simulink model "Marine_LocoMotive_UAV_est_git"  (R2018a)
settings: Solver=ode4  StartTime=0.0  StopTime=40  FixedStep=T  MaxStep=2*T  MinStep=T  RelTol=1e-4
values from neighbouring files (symbols this model uses):
  a_11 = 0.05*m_b    (= 0.625)    [Marine_LocoMotive_UAV_est_git_parameters.m]    (also in Marine_LocoMotive_UAV_medium_est_git_parameters.m = 1.6875; heave_dynamics_chart.m)
  a_33 = m_b    (= 12.5)    [Marine_LocoMotive_UAV_est_git_parameters.m]    (also in Marine_LocoMotive_UAV_medium_est_git_parameters.m = 33.75; heave_dynamics_chart.m)
  A_w = 1*3.3/2    (= 1.65)    [Marine_LocoMotive_UAV_est_git_parameters.m]    (also in Marine_LocoMotive_UAV_medium_est_git_parameters.m = 0.6)
  A_w2 = 1*1.2/2    (= 0.6)    [Marine_LocoMotive_UAV_est_git_parameters.m]    (also in Marine_LocoMotive_UAV_medium_est_git_parameters.m = 0.305)
  Ac = 0.0331    [Marine_LocoMotive_UAV_est_git_parameters.m]    (also in Marine_LocoMotive_UAV_medium_est_git_parameters.m = 0.422)
  alpha_bar = pi/4    (= 0.785398163397)    [Marine_LocoMotive_UAV_est_git_parameters.m]    (also in Marine_LocoMotive_UAV_medium_est_git_parameters.m; heave_dynamics_chart.m = pi/4*sign(V_bar(j)))
  Am = sysd.denominator{1}    [Marine_LocoMotive_UAV_est_git_parameters.m]    (also in Marine_LocoMotive_UAV_medium_est_git_parameters.m)
  Am1_LPF = sysd.denominator{1}    [Marine_LocoMotive_UAV_est_git_parameters.m]    (also in Marine_LocoMotive_UAV_medium_est_git_parameters.m)
  Am2_LPF = sysd.denominator{1}    [Marine_LocoMotive_UAV_est_git_parameters.m]    (also in Marine_LocoMotive_UAV_medium_est_git_parameters.m)
  Am_asw_LPF = sysd.denominator{1}    [Marine_LocoMotive_UAV_est_git_parameters.m]    (also in Marine_LocoMotive_UAV_medium_est_git_parameters.m)
  Am_coup_LPF = sysd.denominator{1}    [Marine_LocoMotive_UAV_est_git_parameters.m]    (also in Marine_LocoMotive_UAV_medium_est_git_parameters.m)
  Am_fast_coup_LPF = sysd.denominator{1}    [Marine_LocoMotive_UAV_est_git_parameters.m]    (also in Marine_LocoMotive_UAV_medium_est_git_parameters.m)
  Am_rdeL_LPF = sysd.denominator{1}    [Marine_LocoMotive_UAV_est_git_parameters.m]    (also in Marine_LocoMotive_UAV_medium_est_git_parameters.m)
  Am_reL_LPF = sysd.denominator{1}    [Marine_LocoMotive_UAV_est_git_parameters.m]    (also in Marine_LocoMotive_UAV_medium_est_git_parameters.m)
  Am_rref20_LPF = sysd.denominator{1}    [Marine_LocoMotive_UAV_est_git_parameters.m]    (also in Marine_LocoMotive_UAV_medium_est_git_parameters.m)
  Am_rref_LPF = sysd.denominator{1}    [Marine_LocoMotive_UAV_est_git_parameters.m]    (also in Marine_LocoMotive_UAV_medium_est_git_parameters.m)
  AmAlpha_LPF = sysd.denominator{1}    [Marine_LocoMotive_UAV_est_git_parameters.m]    (also in Marine_LocoMotive_UAV_medium_est_git_parameters.m)
  Amp_sf = 3    [Marine_LocoMotive_UAV_est_git_parameters.m]    (also in Marine_LocoMotive_UAV_medium_est_git_parameters.m)
  Amp_sf_rp = 0.05*m_u*g    (= 0.8829)    [Marine_LocoMotive_UAV_est_git_parameters.m]    (also in Marine_LocoMotive_UAV_medium_est_git_parameters.m = 9.56475)
  AmV_LPF = sysd.denominator{1}    [Marine_LocoMotive_UAV_est_git_parameters.m]    (also in Marine_LocoMotive_UAV_medium_est_git_parameters.m)
  AmZ_LPF = sysd.denominator{1}    [Marine_LocoMotive_UAV_est_git_parameters.m]    (also in Marine_LocoMotive_UAV_medium_est_git_parameters.m)
  b_11 = 0    [Marine_LocoMotive_UAV_est_git_parameters.m]    (also in Marine_LocoMotive_UAV_medium_est_git_parameters.m; heave_dynamics_chart.m)
  b_33 = 2*m_b*omega_h    (= 19.6349540849)    [Marine_LocoMotive_UAV_est_git_parameters.m]    (also in Marine_LocoMotive_UAV_medium_est_git_parameters.m = 84.8230016469; buoyancy_calc.m = 4.18879020479; heave_dynamics_chart.m = 2*m_b*omega_h)
  Bm = sysd.numerator{1}    [Marine_LocoMotive_UAV_est_git_parameters.m]    (also in Marine_LocoMotive_UAV_medium_est_git_parameters.m)
  Bm1_LPF = sysd.numerator{1}    [Marine_LocoMotive_UAV_est_git_parameters.m]    (also in Marine_LocoMotive_UAV_medium_est_git_parameters.m)
  Bm2_LPF = sysd.numerator{1}    [Marine_LocoMotive_UAV_est_git_parameters.m]    (also in Marine_LocoMotive_UAV_medium_est_git_parameters.m)
  Bm_asw_LPF = sysd.numerator{1}    [Marine_LocoMotive_UAV_est_git_parameters.m]    (also in Marine_LocoMotive_UAV_medium_est_git_parameters.m)
  Bm_coup_LPF = sysd.numerator{1}    [Marine_LocoMotive_UAV_est_git_parameters.m]    (also in Marine_LocoMotive_UAV_medium_est_git_parameters.m)
  Bm_fast_coup_LPF = sysd.numerator{1}    [Marine_LocoMotive_UAV_est_git_parameters.m]    (also in Marine_LocoMotive_UAV_medium_est_git_parameters.m)
  Bm_rdeL_LPF = sysd.numerator{1}    [Marine_LocoMotive_UAV_est_git_parameters.m]    (also in Marine_LocoMotive_UAV_medium_est_git_parameters.m)
  Bm_reL_LPF = sysd.numerator{1}    [Marine_LocoMotive_UAV_est_git_parameters.m]    (also in Marine_LocoMotive_UAV_medium_est_git_parameters.m)
  Bm_rref20_LPF = sysd.numerator{1}    [Marine_LocoMotive_UAV_est_git_parameters.m]    (also in Marine_LocoMotive_UAV_medium_est_git_parameters.m)
  Bm_rref_LPF = sysd.numerator{1}    [Marine_LocoMotive_UAV_est_git_parameters.m]    (also in Marine_LocoMotive_UAV_medium_est_git_parameters.m)
  BmAlpha_LPF = sysd.numerator{1}    [Marine_LocoMotive_UAV_est_git_parameters.m]    (also in Marine_LocoMotive_UAV_medium_est_git_parameters.m)
  BmV_LPF = sysd.numerator{1}    [Marine_LocoMotive_UAV_est_git_parameters.m]    (also in Marine_LocoMotive_UAV_medium_est_git_parameters.m)
  BmZ_LPF = sysd.numerator{1}    [Marine_LocoMotive_UAV_est_git_parameters.m]    (also in Marine_LocoMotive_UAV_medium_est_git_parameters.m)
  C_S = [5;9]*10^-3    [Marine_LocoMotive_UAV_est_git_parameters.m]    (also in Marine_LocoMotive_UAV_medium_est_git_parameters.m; heave_dynamics_chart.m = 0.075/(log10(Re)-2)^2)
  Cd_u = 0.2    [Marine_LocoMotive_UAV_est_git_parameters.m]    (also in Marine_LocoMotive_UAV_medium_est_git_parameters.m)
  D_x = b_11 + D_s(1)    [Marine_LocoMotive_UAV_est_git_parameters.m]    (also in Marine_LocoMotive_UAV_medium_est_git_parameters.m; heave_dynamics_chart.m = b_11 + D_s(i,j))
  D_z = b_33 + D_s(2)    [Marine_LocoMotive_UAV_est_git_parameters.m]    (also in Marine_LocoMotive_UAV_medium_est_git_parameters.m; heave_dynamics_chart.m)
  dc_M_p = 6.7    [Marine_LocoMotive_UAV_est_git_parameters.m]    (also in Marine_LocoMotive_UAV_medium_est_git_parameters.m)
  Delta_h = (A_im/A_b-0.5)*h_b    (= -0.0625)    [Marine_LocoMotive_UAV_est_git_parameters.m]    (also in Marine_LocoMotive_UAV_medium_est_git_parameters.m = -0.075; heave_dynamics_chart.m)
  eps_V = 0.1    [Marine_LocoMotive_UAV_est_git_parameters.m]    (also in Marine_LocoMotive_UAV_medium_est_git_parameters.m)
  epsilon_1 = 5    [Marine_LocoMotive_UAV_est_git_parameters.m]    (also in Marine_LocoMotive_UAV_medium_est_git_parameters.m)
  epsilon_e_u1 = 0.05    [Marine_LocoMotive_UAV_est_git_parameters.m]    (also in Marine_LocoMotive_UAV_medium_est_git_parameters.m)
  epsilon_w = 0    [Marine_LocoMotive_UAV_est_git_parameters.m]    (also in Marine_LocoMotive_UAV_medium_est_git_parameters.m)
  epsilon_w2 = pi    (= 3.14159265359)    [Marine_LocoMotive_UAV_est_git_parameters.m]    (also in Marine_LocoMotive_UAV_medium_est_git_parameters.m)
  g = 9.81    [Marine_LocoMotive_UAV_est_git_parameters.m]    (also in Marine_LocoMotive_UAV_medium_est_git_parameters.m; heave_dynamics_chart.m)
  gamma_d_p = (2*0.3/0.03*2*0.2*12/4)/10    (= 2.4)    [Marine_LocoMotive_UAV_est_git_parameters.m]    (also in Marine_LocoMotive_UAV_medium_est_git_parameters.m)
  H = 10    [Marine_LocoMotive_UAV_est_git_parameters.m]    (also in Marine_LocoMotive_UAV_medium_est_git_parameters.m)
  h_b = 0.25    [Marine_LocoMotive_UAV_est_git_parameters.m]    (also in Marine_LocoMotive_UAV_medium_est_git_parameters.m = 0.3; buoyancy_calc.m = 0.15; heave_dynamics_chart.m)
  J_b = m_b*h_b*l_b/12    (= 0.208333333333)    [Marine_LocoMotive_UAV_est_git_parameters.m]    (also in Marine_LocoMotive_UAV_medium_est_git_parameters.m = 1.265625; heave_dynamics_chart.m)
  J_u = 0.03    [Marine_LocoMotive_UAV_est_git_parameters.m]    (also in Marine_LocoMotive_UAV_medium_est_git_parameters.m = 1.51708333333)
  K = 40    [Marine_LocoMotive_UAV_est_git_parameters.m]    (also in Marine_LocoMotive_UAV_medium_est_git_parameters.m = 83.3333333333)
  k3 = 24    [Marine_LocoMotive_UAV_est_git_parameters.m]    (also in Marine_LocoMotive_UAV_medium_est_git_parameters.m)
  k4 = 0.8    [Marine_LocoMotive_UAV_est_git_parameters.m]    (also in Marine_LocoMotive_UAV_medium_est_git_parameters.m)
  k_w = omega_w^2/g    (= 0.0628797426165)    [Marine_LocoMotive_UAV_est_git_parameters.m]    (also in Marine_LocoMotive_UAV_medium_est_git_parameters.m = 0.160972141098; heave_dynamics_chart.m = omega_w^2/g)
  k_w2 = omega_w2^2/g    (= 0.160972141098)    [Marine_LocoMotive_UAV_est_git_parameters.m]    (also in Marine_LocoMotive_UAV_medium_est_git_parameters.m = 0.251518970466)
  kd_a = 5.6    [Marine_LocoMotive_UAV_est_git_parameters.m]    (also in Marine_LocoMotive_UAV_medium_est_git_parameters.m)
  kd_r = 19.5    [Marine_LocoMotive_UAV_est_git_parameters.m]    (also in Marine_LocoMotive_UAV_medium_est_git_parameters.m)
  kd_t = 10    [Marine_LocoMotive_UAV_est_git_parameters.m]    (also in Marine_LocoMotive_UAV_medium_est_git_parameters.m = 25)
  kd_x = 5    [Marine_LocoMotive_UAV_est_git_parameters.m]    (also in Marine_LocoMotive_UAV_medium_est_git_parameters.m)
  kd_z = 2    [Marine_LocoMotive_UAV_est_git_parameters.m]    (also in Marine_LocoMotive_UAV_medium_est_git_parameters.m)
  ki_a = 1.6    [Marine_LocoMotive_UAV_est_git_parameters.m]    (also in Marine_LocoMotive_UAV_medium_est_git_parameters.m)
  ki_r = 9    [Marine_LocoMotive_UAV_est_git_parameters.m]    (also in Marine_LocoMotive_UAV_medium_est_git_parameters.m)
  ki_T = 12    [Marine_LocoMotive_UAV_est_git_parameters.m]    (also in Marine_LocoMotive_UAV_medium_est_git_parameters.m)
  ki_x = 1.2    [Marine_LocoMotive_UAV_est_git_parameters.m]    (also in Marine_LocoMotive_UAV_medium_est_git_parameters.m)
  ki_z = 1    [Marine_LocoMotive_UAV_est_git_parameters.m]    (also in Marine_LocoMotive_UAV_medium_est_git_parameters.m)
  kp_a = 9.6    [Marine_LocoMotive_UAV_est_git_parameters.m]    (also in Marine_LocoMotive_UAV_medium_est_git_parameters.m)
  kp_r = 45    [Marine_LocoMotive_UAV_est_git_parameters.m]    (also in Marine_LocoMotive_UAV_medium_est_git_parameters.m)
  kp_t = 20    [Marine_LocoMotive_UAV_est_git_parameters.m]    (also in Marine_LocoMotive_UAV_medium_est_git_parameters.m = 50)
  kp_T = 25    [Marine_LocoMotive_UAV_est_git_parameters.m]    (also in Marine_LocoMotive_UAV_medium_est_git_parameters.m)
  kp_x = 7    [Marine_LocoMotive_UAV_est_git_parameters.m]    (also in Marine_LocoMotive_UAV_medium_est_git_parameters.m)
  kp_z = 3    [Marine_LocoMotive_UAV_est_git_parameters.m]    (also in Marine_LocoMotive_UAV_medium_est_git_parameters.m)
  L = 0.2    [Marine_LocoMotive_UAV_est_git_parameters.m]    (also in Marine_LocoMotive_UAV_medium_est_git_parameters.m = 0.8)
  l_b = 0.8    [Marine_LocoMotive_UAV_est_git_parameters.m]    (also in Marine_LocoMotive_UAV_medium_est_git_parameters.m = 1.5; buoyancy_calc.m = 0.5; heave_dynamics_chart.m)
  Lc_0 = 7    [Marine_LocoMotive_UAV_est_git_parameters.m]    (also in Marine_LocoMotive_UAV_medium_est_git_parameters.m = 20)
  LIMIT_CMD_PITCH = 45*pi/180    (= 0.785398163397)    [Marine_LocoMotive_UAV_est_git_parameters.m]    (also in Marine_LocoMotive_UAV_medium_est_git_parameters.m)
  LIMIT_uCMD_HEIGHT = 0.9*n_motors*K    (= 144)    [Marine_LocoMotive_UAV_est_git_parameters.m]    (also in Marine_LocoMotive_UAV_medium_est_git_parameters.m = 450)
  m_b = rho_w*Vol_b/4    (= 12.5)    [Marine_LocoMotive_UAV_est_git_parameters.m]    (also in Marine_LocoMotive_UAV_medium_est_git_parameters.m = 33.75; buoyancy_calc.m = 5; heave_dynamics_chart.m)
  m_u = 1.8    [Marine_LocoMotive_UAV_est_git_parameters.m]    (also in Marine_LocoMotive_UAV_medium_est_git_parameters.m = 19.5)
  min_sf = 5    [Marine_LocoMotive_UAV_est_git_parameters.m]    (also in Marine_LocoMotive_UAV_medium_est_git_parameters.m)
  min_sf_rp = 0.35*m_u*g    (= 6.1803)    [Marine_LocoMotive_UAV_est_git_parameters.m]    (also in Marine_LocoMotive_UAV_medium_est_git_parameters.m = 66.95325)
  n_motors = 4    [Marine_LocoMotive_UAV_est_git_parameters.m]    (also in Marine_LocoMotive_UAV_medium_est_git_parameters.m = 6)
  nu_w = 1.787*10^-6    (= 1.787e-06)    [Marine_LocoMotive_UAV_est_git_parameters.m]    (also in Marine_LocoMotive_UAV_medium_est_git_parameters.m; buoyancy_calc.m; heave_dynamics_chart.m)
  omega_w = 2*pi/T_w    (= 0.785398163397)    [Marine_LocoMotive_UAV_est_git_parameters.m]    (also in Marine_LocoMotive_UAV_medium_est_git_parameters.m = 1.25663706144; heave_dynamics_chart.m = 2*pi/T_i)
  omega_w2 = 2*pi/T_w2    (= 1.25663706144)    [Marine_LocoMotive_UAV_est_git_parameters.m]    (also in Marine_LocoMotive_UAV_medium_est_git_parameters.m = 1.57079632679)
  r_0 = sqrt( (X0_b(1) - X0_u(1))^2 +(X0_b(2) - X0_u(2))^2 )    [Marine_LocoMotive_UAV_est_git_parameters.m]    (also in Marine_LocoMotive_UAV_medium_est_git_parameters.m)
  R_b = 0.1    [buoyancy_calc.m]
  r_bar = Lc_0-0.3    (= 6.7)    [Marine_LocoMotive_UAV_est_git_parameters.m]    (also in Marine_LocoMotive_UAV_medium_est_git_parameters.m = 19.7)
  r_min = (zu_bar-H)-0.2    [Marine_LocoMotive_UAV_est_git_parameters.m]    (also in Marine_LocoMotive_UAV_medium_est_git_parameters.m)
  rho_a = 1.225    [Marine_LocoMotive_UAV_est_git_parameters.m]    (also in Marine_LocoMotive_UAV_medium_est_git_parameters.m)
  rho_w = 1000    [Marine_LocoMotive_UAV_est_git_parameters.m]    (also in Marine_LocoMotive_UAV_medium_est_git_parameters.m; buoyancy_calc.m; heave_dynamics_chart.m)
  T = 1/500    (= 0.002)    [Marine_LocoMotive_UAV_est_git_parameters.m]    (also in Marine_LocoMotive_UAV_medium_est_git_parameters.m)
  T_init = 10    [Marine_LocoMotive_UAV_est_git_parameters.m]    (also in Marine_LocoMotive_UAV_medium_est_git_parameters.m)
  Theta0 = 0    [Marine_LocoMotive_UAV_est_git_parameters.m]    (also in Marine_LocoMotive_UAV_medium_est_git_parameters.m)
  torque_corr = 2*cosd(60)+1    [Marine_LocoMotive_UAV_est_git_parameters.m]    (also in Marine_LocoMotive_UAV_medium_est_git_parameters.m)
  u_s = w_dir*A_w^2*omega_w*k_w*exp(2*k_w*(-Delta_h/2))    [Marine_LocoMotive_UAV_est_git_parameters.m]    (also in Marine_LocoMotive_UAV_medium_est_git_parameters.m)
  u_s2 = w_dir2*A_w2^2*omega_w2*k_w2*exp(2*k_w2*(-Delta_h/2))    [Marine_LocoMotive_UAV_est_git_parameters.m]    (also in Marine_LocoMotive_UAV_medium_est_git_parameters.m)
  u_t = -1*0.5*1    (= -0.5)    [Marine_LocoMotive_UAV_est_git_parameters.m]    (also in Marine_LocoMotive_UAV_medium_est_git_parameters.m)
  u_w = 0*0.2    (= 0)    [Marine_LocoMotive_UAV_est_git_parameters.m]    (also in Marine_LocoMotive_UAV_medium_est_git_parameters.m)
  V0_b = [u_t+u_w+u_s+v_x_w, v_z_w].*[1 1]    [Marine_LocoMotive_UAV_est_git_parameters.m]    (also in Marine_LocoMotive_UAV_medium_est_git_parameters.m = [u_t+u_w+u_s+v_x_w, v_z_w])
  V0_u = V0_b    [Marine_LocoMotive_UAV_est_git_parameters.m]    (also in Marine_LocoMotive_UAV_medium_est_git_parameters.m = [0 0])
  V_bar = 4    [Marine_LocoMotive_UAV_est_git_parameters.m]    (also in Marine_LocoMotive_UAV_medium_est_git_parameters.m; heave_dynamics_chart.m = [-20:0.1:20]')
  Vol_b = A_b*l_b    (= 0.05)    [Marine_LocoMotive_UAV_est_git_parameters.m]    (also in Marine_LocoMotive_UAV_medium_est_git_parameters.m = 0.135; heave_dynamics_chart.m)
  w_dir = 1    [Marine_LocoMotive_UAV_est_git_parameters.m]    (also in Marine_LocoMotive_UAV_medium_est_git_parameters.m; heave_dynamics_chart.m)
  w_dir2 = 1    [Marine_LocoMotive_UAV_est_git_parameters.m]    (also in Marine_LocoMotive_UAV_medium_est_git_parameters.m)
  X0_b = [0,H-Delta_h]    [Marine_LocoMotive_UAV_est_git_parameters.m]    (also in Marine_LocoMotive_UAV_medium_est_git_parameters.m)
  X0_u = X0_b + [3/7 3/7]*Lc_0    [Marine_LocoMotive_UAV_est_git_parameters.m]    (also in Marine_LocoMotive_UAV_medium_est_git_parameters.m)
  zu_bar = X0_b(2) + Lc_0*sin(alpha_bar_0)    [Marine_LocoMotive_UAV_est_git_parameters.m]    (also in Marine_LocoMotive_UAV_medium_est_git_parameters.m)
undefined symbols (not defined in the file or in its folder): Am_HPF, Am_LPF, Am_LPF2, an1, an1_v, an2, an3, Bm_HPF, Bm_LPF, Bm_LPF2, bn1, bn1_v, bn2, bn3, DiscIntNeverNeededParam, F, Light, magnitude, MIL, OMEGA_FILTER_OUTER, Tc, Tg, Tn, Ts, Tsc, Tz, X_GPS_offset
libraries: simulink x55, simulink_extras x9, aerolibwind2 x2
(part 9 of 9)

== matlab function Marine_LocoMotive_UAV_est_git/UAV controller/State Machine new ==
  settings: updateMethod=DISCRETE  sampleTime=T
  data: eps input; r input; r_thr input; active output; decelerate output; switch_side output; xdot_b input; V_bar0 input; c output; V_bar input; V_bar_dot input; alpha input; alpha_bar input; x_rel_final input; x_rel input; reset input
function [active,decelerate,switch_side,c] = fcn(eps,r, r_thr, ...
    xdot_b, V_bar0, V_bar, V_bar_dot, alpha, alpha_bar, x_rel_final, x_rel...
    , reset)

persistent state
persistent is_active
persistent decelerating
persistent switching_side

if isempty(is_active) 
    state = 0;
    is_active = 0;
    decelerating = 0;
    switching_side = 0;
end

eps = abs(eps); % make sure that eps is positive.
eps_p1 = 2*eps;
eps_p2 = 2.5*eps;
eps_n1 = 1.5*eps;
eps_n2 = 2*eps;

dx_thr = 0.13;  
% deactivate the velocity controller while reset is on:
if (reset == 1)
    is_active = 0;
    decelerating = 0;
    switching_side = 0;
    % idel state
    state = 0; 
% buoy velocity is low, activate to accelerate:
elseif and( is_active == 0 && decelerating == 0 && switching_side == 0,...
        and( xdot_b <= V_bar0-eps_n1, alpha < pi/2 ) ) 
    is_active = 1;
    % accelerate flag state
    state = 1;     
% % keep activated while pursuing the desired velocity    
% elseif and( is_active == 1 && decelerating == 0 && switching_side == 0 && V_bar_dot >= 0,...
%         and( xdot_b < V_bar+eps_p1, alpha < pi/2 ) ) 
%     is_active = 1;
%     decelerating = 0; 
%     switching_side = 0;
%     % accelerating state
%     c = 2; 
% elseif and( is_active == 1 && decelerating == 0 && switching_side == 0 && V_bar_dot < 0,...,...
%         and( xdot_b < V_bar+eps_n1, alpha < pi/2 ) ) 
%     is_active = 1;
%     decelerating = 0; 
%     switching_side = 0;
%     % accelerating state
%     c = 2.5;     
% deactivate since velocity has gone too high or the system has
% unintentionnally decouple to prevent damage (removed for testing):
elseif and( is_active == 1 && decelerating == 0 && switching_side == 0 && V_bar_dot >= 0,...
        or( (xdot_b >= V_bar+eps_p1), 0 )) % (r < r_thr)
    is_active = 0;
    % acceleration stop state
    state = 2;
elseif and( is_active == 1 && decelerating == 0 && switching_side == 0 && V_bar_dot < 0,...
        or( (xdot_b >= V_bar+eps_n1), (r < r_thr) )) % (r < r_thr)
    is_active = 0;
    % acceleration stop state
    state = 3;    
% % keep deactivated since velocity error has not reached the 
% % upper and lower thresholds:    
% elseif and( is_active==0  && decelerating==0 && switching_side==0 && alpha<pi/2 && V_bar_dot >= 0,...
%         and(xdot_b > V_bar-eps_n1 , xdot_b < V_bar+eps_p2 ) ) 
%     is_active = 0;
%     decelerating = 0; 
%     switching_side = 0;
%     % forward elevation-hold state
%     c = 4;
% elseif and( is_active==0  && decelerating==0 && switching_side==0 && alpha<pi/2 && V_bar_dot < 0,...
%         and(xdot_b > V_bar-eps_n1 , xdot_b < V_bar+0.6*eps_n1 ) ) 
%     is_active = 0;
%     decelerating = 0; 
%     switching_side = 0;
%     % forward elevation-hold state
%     c = 4.5;    
% % prepare to decelerate since velocity is too high:    
% elseif and( is_active == 0  && decelerating == 0 && switching_side == 0 && V_bar_dot >= 0,...
%         and( xdot_b >= V_bar0+eps_p2, alpha < pi/2 ) )  
%     is_active = 0;
%     decelerating = 1; 
%     switching_side = 0;
%     % decelerate flag state
%     c = 5;     
% elseif and( is_active == 0  && decelerating == 0 && switching_side == 0 && V_bar_dot < 0,...
%         and( xdot_b >= V_bar0+0.6*eps_n1, alpha < pi/2 ) )  
%     is_active = 0;
%     decelerating = 1; 
%     switching_side = 0;
%     % decelerate flag state
%     c = 5.5;    
% declare UAV switching side state:    
elseif and( is_active == 0 && decelerating == 0 && switching_side == 0 && V_bar_dot < 0,...
         and( xdot_b > V_bar0+eps_n1 , alpha_bar < pi/2 ) )
    decelerating = 1;
    switching_side = 1;
    % switch side flag state
    state = 4;     
% % move the UAV to the other side of the buoy to be able to decelerate:    
% elseif and( is_active == 0 && decelerating == 0 && switching_side == 0,...
%         not(and(abs(x_rel-x_rel_final) <= 0.05, alpha_bar > pi/2) ))
% %        not(and(abs(alpha-alpha_bar_step) <= 0.5*(pi/180), alpha_bar > pi/2) ))
%     is_active = 0;
%     decelerating = 1; 
%     switching_side = 1;
%     % switching side state
%     c = 7; 
% Stop switching side and prepare to return to elevation hold with (alpha > pi/2):    
elseif and( is_active == 0 && decelerating == 1 && switching_side == 1,...
         and(abs(x_rel-x_rel_final) <= dx_thr, alpha_bar > pi/2  ))
    % and(abs(alpha_bar_step-alpha_bar_switch) <= 1*(pi/180) ,...
    switching_side = 0;
    % switching side stop state
    state = 5;
% activate deceleration action (alpha > pi/2):    
elseif and( is_active == 0 && decelerating == 1 && switching_side == 0,...
         and(alpha_bar > pi/2 , xdot_b > V_bar0+eps_n1 )  )
    is_active = 1;
    % switching side stop state
    state = 6;  
% % Keep deceleration:    
% elseif and( is_active == 1 && decelerating == 1 && switching_side == 0,...
%         and(alpha_bar > pi/2 , xdot_b > V_bar0-eps_p1 )  )
%     is_active = 1;
%     decelerating = 1; 
%     switching_side = 0;    
%     c = 10;    
% stop decelerating after velocity error is reduced ...
% or if the system has decoupled (removed for testing):    
elseif and( is_active == 1 && decelerating == 1 && switching_side == 0,...
        and(alpha_bar > pi/2 , or( (xdot_b <= V_bar0-eps_p1), 0 ))) % (r < r_thr)
    is_active = 0;
    state = 7;
% % keep deactivated since velocity error has not reached the threshold:    
% elseif and( is_active==0  && decelerating==1 && switching_side==0 && alpha>pi/2,...
%         and( xdot_b < V_bar0+eps_n1 , xdot_b > V_bar0-eps_p2 ) ) 
%     is_active = 0;
%     decelerating = 1; 
%     switching_side = 0;
%     % backwark elevation-hold state
%     c = 12;     
% prepare to accelerate since velocity is too low:    
elseif and( is_active == 0  && decelerating == 1 && switching_side == 0,...
        and( xdot_b < V_bar0-eps_p2 , alpha > pi/2 ) ) 
    decelerating = 0; 
    % accelerate flag state
    state = 8;      
% declare UAV switching side state (to forward):    
elseif and( is_active == 0 && decelerating == 0 && switching_side == 0,...
         and( xdot_b < V_bar0-eps_p1 , alpha_bar > pi/2 ) )
     switching_side = 1;
    % switch side flag state
    state = 9;     
% % move the UAV to the other (front) side of the buoy to be able to decelerate:    
% elseif and( is_active == 0 && decelerating == 0 && switching_side == 1,...
%         not(and(abs(alpha-alpha_bar) <= 1*(pi/180), alpha_bar < pi/2) ))
%     is_active = 0;
%     decelerating = 0; 
%     switching_side = 1;
%     % switching side state
%     c = 15; 
% Stop switching side and prepare to return to elevation hold with (alpha < pi/2):    
elseif and( is_active == 0 && decelerating == 0 && switching_side == 1,...
         and(abs(x_rel-x_rel_final) <= dx_thr, alpha_bar < pi/2)  )    
    switching_side = 0;
    % switching side stop state
    state = 10;    
% need completion for other cases (to switch from backward to forward motion)...    
end    

    
%%
c           = state;
active      =  is_active;
decelerate  =  decelerating;   
switch_side =  switching_side;

== matlab function Marine_LocoMotive_UAV_est_git/UAV controller/Coupling /u_T switch/MATLAB Function ==
  data: u_T input; u_T_out output; alpha input; theta_u input; m_q input; g input; c output
function [u_T_out,c] = fcn(u_T, alpha, theta_u, m_q, g)

threshold = m_q*g*sin(alpha);
c = 0;
if alpha <= pi/2
    if u_T <= threshold
        if (alpha + theta_u) >= 0
            u_T_out = max(u_T, threshold);
            c = 1;
        else
            u_T_out = u_T;
        end
    else 
        if (alpha + theta_u) < 0
            u_T_out = 0;
            c = 1;
        else 
            u_T_out = u_T;
        end
    end
    
else % alpha > pi/2
    if u_T < threshold
        if (alpha + theta_u) < pi
            u_T_out = max(u_T, threshold);
            c = 1;
        else
            u_T_out = u_T;
        end
    else 
        if (alpha + theta_u) < pi
            u_T_out = u_T;           
        else 
            u_T_out = 0;
            c = 1;
        end
    end    
end

== matlab function Marine_LocoMotive_UAV_est_git/UAV controller/Coupling /Subsystem3/MATLAB Function ==
  data: u_T input; u_T_out output; alpha input; theta_u input; m_q input; g input; c output
function [u_T_out,c] = fcn(u_T, alpha, theta_u, m_q, g)

threshold = m_q*g*sin(alpha);
c = 0;
if alpha <= pi/2
    if u_T <= threshold
        if (alpha + theta_u) >= 0
            u_T_out = min(u_T, threshold);
            c = 1;
        else
            u_T_out = u_T;
        end
    else 
        if (alpha + theta_u) < 0
            u_T_out = 0;
            c = 1;
        else 
            u_T_out = u_T;
        end
    end
    
else % alpha > pi/2
    if u_T < threshold
        if (alpha + theta_u) < pi
            u_T_out = min(u_T, threshold);
            c = 1;
        else
            u_T_out = u_T;
        end
    else 
        if (alpha + theta_u) < pi
            u_T_out = u_T;           
        else 
            u_T_out = 0;
            c = 1;
        end
    end    
end

== matlab function Marine_LocoMotive_UAV_est_git/Sensors and Filters/Data processing/Estimate Attitude/Calculate Roll and Pitch (From Acceleration Data)/calc_roll_pitch ==
  data: roll_acc output; pitch_acc output; acc_body input
function [roll_acc, pitch_acc]   = fcn(acc_body)
%#eml
n = norm(acc_body,2);
if n>eps
    acc_body = -acc_body/n; 
else
    acc_body = [0 0 1]';
end

roll_acc = atan2(acc_body(2),acc_body(3));
pitch_acc = atan2( -acc_body(1), acc_body(2)*sin(roll_acc)+acc_body(3)*cos(roll_acc));

== matlab function Marine_LocoMotive_UAV_est_git/Sensors and Filters/Data processing/Estimate Position/Kalman Filter - Height ==
  settings: updateMethod=DISCRETE  sampleTime=T
  data: height output; optitrack input; sonar_d input; dt input; x0 input
function height   = fcn(optitrack,sonar_d,dt,x0)
%#eml

     Q_sonar  = 0.1; %0.01; %0.001
     Q_optitrack   = 0.01; %0.01;  %0.003
     R_height =  0.03;  %0.03

    
    persistent P_00;
    persistent P_01;
    persistent P_10;
    persistent P_11;
    persistent x_height;
    persistent x_bias;
        
    if isempty(P_00)
        P_00 = 0;
    end
    
    if isempty(P_01)
        P_01 = 0;
    end
    if isempty(P_10)
        P_10 = 0;
    end
    if isempty(P_11)
        P_11 = 0;
    end
    if isempty(x_bias)
       x_bias = 0;
    end
    if isempty(x_height)
       x_height = x0;
    end
    
    
    % Compensate for sonar rate calculation (sonar sample rate is 10Hz)
    sonar_d_corrected = sonar_d*dt*10;  % m/s
    
    % Reject large height rate changes from sonar
    % As those are likely a result of obstacle underneath or noise
    if(abs(sonar_d_corrected) > 1 )    % max height rate (m/s)
        sonar_d_corrected = 0;
    end
    
    % Calculate the new output
    %x_height = x_height + dt * (sonar_d - x_bias); % old 
    x_height = x_height + dt * (sonar_d_corrected - x_bias);
    P_00 = P_00 -  dt * (P_10 + P_01) + Q_sonar * dt;
    P_01 = P_01  - dt * P_11;
    P_10 = P_10  - dt * P_11;
    P_11 = P_11  + Q_optitrack * dt;

    % Assuming H = [0.95 (effect of optitrack) 0.05 (effect of sonar)]
    e = (0.05*x_height + 0.95*optitrack) - x_height;
    S = P_00 + R_height;
    K_0 = P_00 / S;
    K_1 = P_10 / S;

    % Correction
    x_height = x_height+  K_0 * e;
    x_bias  = x_bias+  K_1 * e;
    P_00 = P_00 - K_0 * P_00;
    P_01 = P_01 - K_0 * P_01;
    P_10 = P_10 - K_1 * P_00;
    P_11 = P_11 - K_1 * P_01;

    height = x_height;
